simulink model "Masa_Resorte_Duro (jose-OptiPlex-7460-AIO_s conflicted copy 2019-10-16)"  (R2018b)
settings: Solver=ode45  StartTime=0.0  StopTime=500  MaxStep=0.01  RelTol=1e-3  EnableMultiTasking=on
values from neighbouring files (symbols this model uses):
  a = 15    [Data20_Sept_2019 (jose-OptiPlex-7460-AIO_s conflicted copy 2019-10-16).mat]    (also in Masa_Resorte_Duro_Parametros.m)
  B = 0.5    [Data20_Sept_2019 (jose-OptiPlex-7460-AIO_s conflicted copy 2019-10-16).mat]    (also in Masa_Resorte_Duro_Parametros.m)
  Ci1 = 0    [Data20_Sept_2019 (jose-OptiPlex-7460-AIO_s conflicted copy 2019-10-16).mat]    (also in Masa_Resorte_Duro_Parametros.m; Pendulo_SNL_Parametros.m = 0.785398163397)
  Ci2 = 0    [Data20_Sept_2019 (jose-OptiPlex-7460-AIO_s conflicted copy 2019-10-16).mat]    (also in Masa_Resorte_Duro_Parametros.m; Pendulo_SNL_Parametros.m)
  k = 0.1    [Data20_Sept_2019 (jose-OptiPlex-7460-AIO_s conflicted copy 2019-10-16).mat]    (also in Masa_Resorte_Duro_Parametros.m; Pendulo_SNL_Parametros.m = 0.5)
  m = 1    [Data20_Sept_2019 (jose-OptiPlex-7460-AIO_s conflicted copy 2019-10-16).mat]    (also in Masa_Resorte_Duro_Parametros.m; Pendulo_SNL_Parametros.m)
settings Model: Creator=Jose  LastModifiedBy=root
settings DataIOCC: LimitDataPoints=on  SaveFormat=Array
settings OptimizationCC: LifeSpan=inf
settings DebuggingCC: SolverPrmCheckMsg=warning  SFUnexpectedBacktrackingDiag=warning  SFNoUnconditionalDefaultTransitionDiag=warning  SFExecutionAtInitializationDiag=none
settings HardwareCC: ProdBitPerPointer=32  ProdBitPerSizeT=32  ProdBitPerPtrDiffT=32  ProdLargestAtomicFloat=None  ProdIntDivRoundTo=Undefined  ProdEndianess=Unspecified  ProdWordSize=32  ProdHWDeviceType=32-bit Generic
settings ModelReferenceCC: PropagateSignalLabelsOutOfModel=off
settings SFSimCC: SimUseLocalCustomCode=off
settings RTWCC: RTWUseLocalCustomCode=off
settings CodeAppCC: StateflowObjectComments=on
settings GRTTargetCC: TargetLangStandard=C89/C90 (ANSI)  GeneratePreprocessorConditionals=Disable all
settings ConfigComp: CovMetricSettings=dw  CovHtmlReporting=on  CovSaveCumulativeToWorkspaceVar=on  CovSaveSingleToWorkspaceVar=on  CovExternalEMLEnable=off  CovSFcnEnable=off

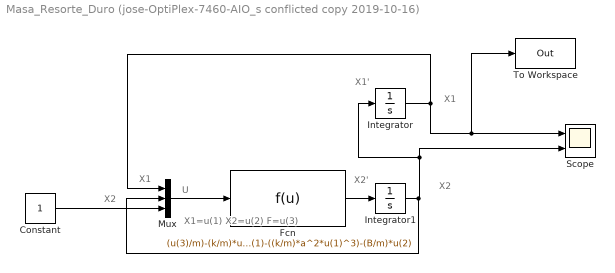
== system Masa_Resorte_Duro (jose-OptiPlex-7460-AIO_s conflicted copy 2019-10-16) ==
  note: X1=u(1)
      | X2=u(2)
      | F=u(3)
  note: U
  note: X2
  note: X1
  note: X2'
  note: X1'
  note: X1
  note: X2
  Constant : Constant
  Fcn : Fcn  Expr=(u(3)/m)-(k/m)*u(1)-((k/m)*a^2*u(1)^3)-(B/m)*u(2)
  Integrator : Integrator  InitialCondition=Ci1
  Integrator1 : Integrator  InitialCondition=Ci2
  Mux : Mux  Inputs=3
  Scope : Scope  NumInputPorts=2
  To Workspace : ToWorkspace  VariableName=Out  SampleTime=0.5
  wires:
  Integrator1/1 -> Mux/2, Scope/2, Integrator/1
  Fcn/1 -> Integrator1/1
  Mux/1 -> Fcn/1
  Integrator/1 -> Mux/1, To Workspace/1, Scope/1
  Constant/1 -> Mux/3
